simulink model "single-phase-grid-connected-inverter"  (R2020a)
settings: Solver=ode45  StartTime=0.0  StopTime=0.1  MaxStep=1e-7  MinStep=1e-8  RelTol=1e-3
libraries: powerlib x15, powerlib_meascontrol x4, simulink x1
settings Model: Creator=LENOVO PC  LastModifiedBy=User
settings SolverCC: ZeroCrossAlgorithm=Adaptive
settings DebuggingCC: IgnoredZcDiagnostic=none

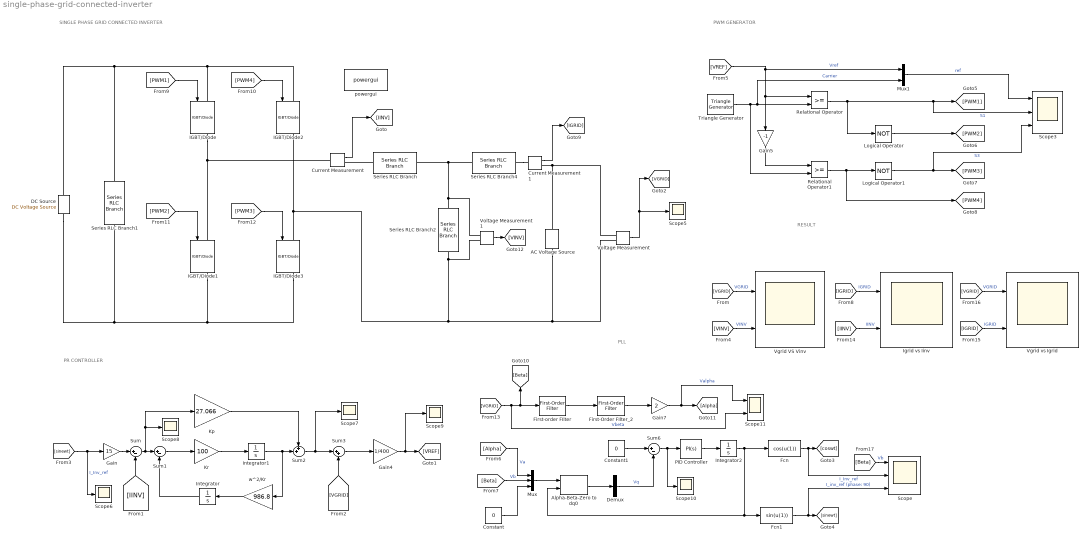
== system single-phase-grid-connected-inverter ==
  note: PR CONTROLLER
  note: SINGLE PHASE GRID CONNECTED INVERTER
  note: PWM GENERATOR
  note: PLL
  note: RESULT
  AC Voltage Source : powerlib/Electrical Sources/AC Voltage Source  Amplitude=325  Phase=0  Frequency=50  SampleTime=0  Measurements=None  BusType=swing  Pref=10e3  Qref=0  Qmin=-inf  Qmax=+inf
  Alpha-Beta-Zero to dq0 : powerlib_meascontrol/Transformations/Alpha-Beta-Zero to dq0  Alignment=90 degrees behind phase A axis
  Constant : Constant  Value=0
  Constant1 : Constant  Value=0
  Current Measurement : powerlib/Measurements/Current Measurement  PhasorSimulation=off  OutputType=Complex  PSBequivalent=0
  Current Measurement1 : powerlib/Measurements/Current Measurement  PhasorSimulation=off  OutputType=Complex  PSBequivalent=0
  DC Source : powerlib/Electrical Sources/DC Voltage Source  Amplitude=400  Measurements=None
  Demux : Demux  Outputs=3
  Fcn : Fcn  Expr=cos(u(1))
  Fcn1 : Fcn  Expr=sin(u(1))
  "First-Order FIlter_2 " : powerlib_meascontrol/Filters/First-Order Filter  FilterType=Lowpass  Tc=1/(2*pi*50)  Ts=0  Initialize=off  Vac_Init=[0, 0, 60]  Vdc_Init=0  PlotResponse=off  FreqRange="[0,  200,  1]"
  First-order FIlter : powerlib_meascontrol/Filters/First-Order Filter  FilterType=Lowpass  Tc=1/(2*pi*50)  Ts=0  Initialize=off  Vac_Init=[0, 0, 60]  Vdc_Init=0  PlotResponse=off  FreqRange="[0,  200,  1]"
  Gain : Gain  Gain=15
  Gain4 : Gain  Gain=1/400
  Gain5 : Gain  Gain=-1
  Gain7 : Gain  Gain=2
  IGBT/Diode{,1..3} (4 alike) : powerlib/Power Electronics/IGBT//Diode  Ron=1e-3  Rs=1e5  Cs=inf  Measurements=on
  Igrid vs Iinv : Scope  NumInputPorts=2
  Integrator : Integrator
  Integrator1 : Integrator
  Integrator2 : Integrator
  Kp : Gain  Gain=27.066
  Kr : Gain  Gain=100
  Logical Operator : Logic  Operator=NOT  Inputs=1  AllPortsSameDT=off  OutDataTypeStr=boolean
  Logical Operator1 : Logic  Operator=NOT  Inputs=1  AllPortsSameDT=off  OutDataTypeStr=boolean
  Mux : Mux  Inputs=3
  Mux1 : Mux  Inputs=2
  PID Controller : simulink/Continuous/PID Controller  Controller=PI  Form=Parallel  TimeDomain=Continuous-time  UseExternalTs=off  SampleTime=-1  IntegratorMethod=Forward Euler  FilterMethod=Forward Euler  ControllerParametersSource=internal  P=10  I=50000  D=0  UseFilter=on  N=100  TunerSelectOption=Transfer Function Based (PID Tuner App)  InitialConditionSource=internal  InitialConditionForIntegrator=0  InitialConditionForFilter=0  DifferentiatorICPrevScaledInput=0  ExternalReset=none  TrackingMode=off  Kt=1  LimitOutput=off  UpperSaturationLimit=inf  LowerSaturationLimit=-inf  LinearizeAsGain=on  AntiWindupMode=none  Kb=1  POutMin=[]  POutMax=[]  IOutMin=[]  IOutMax=[]  DOutMin=[]  DOutMax=[]  NOutMin=[]  NOutMax=[]  SumOutMin=[]  SumOutMax=[]  SaturationOutMin=[]  SaturationOutMax=[]  PParamMin=[]  PParamMax=[]  IParamMin=[]  IParamMax=[]  DParamMin=[]  DParamMax=[]  NParamMin=[]  NParamMax=[]  KbParamMin=[]  KbParamMax=[]  KtParamMin=[]  KtParamMax=[]  KbOutMin=[]  KbOutMax=[]  KtOutMin=[]  KtOutMax=[]  IntegratorOutMin=[]  IntegratorOutMax=[]  FilterOutMin=[]  FilterOutMax=[]  SumI1OutMin=[]  SumI1OutMax=[]  SumI2OutMin=[]  SumI2OutMax=[]  SumI3OutMin=[]  SumI3OutMax=[]  SumI4OutMin=[]  SumI4OutMax=[]  SumDOutMin=[]  SumDOutMax=[]  DifferentiatorOutMin=[]  DifferentiatorOutMax=[]  FilterDiffOutCoefMin=[]  FilterDiffOutCoefMax=[]  ReciprocalOutMin=[]  ReciprocalOutMax=[]  SumDenOutMin=[]  SumDenOutMax=[]  SumNumOutMin=[]  SumNumOutMax=[]  DivideOutMin=[]  DivideOutMax=[]  UdiffTsProdOutMin=[]  UdiffTsProdOutMax=[]  NTsProdOutMin=[]  NTsProdOutMax=[]  UintegralTsProdOutMin=[]  UintegralTsProdOutMax=[]  UngainTsProdOutMin=[]  UngainTsProdOutMax=[]  IntegratorContinuousStateAttributes=''  IntegratorStateMustResolveToSignalObject=off  IntegratorRTWStateStorageClass=Auto  FilterContinuousStateAttributes=''  FilterStateMustResolveToSignalObject=off  FilterRTWStateStorageClass=Auto  ParallelPVariant=InternalParameters  IdealPVariant=Disabled  IVariant=InternalParameters  DVariant=Disabled  IntegratorVariant=Continuous  SatVariant=Disabled  AWVariant=Passthrough  PCopyVariant=Disabled  TRVariant=Disabled  FdbkBlocksVariant=Forward  IdealPFdbkVariant=Disabled  SatFdbkVariant=Disabled  DerivativeFilterVariant=Disabled  NVariant=Disabled  NCopyVariant=Disabled_SignalSpec  FilterICVariant=Disabled  IntegratorICVariant=InternalICs  ExternalResetVariant=Disabled  TRSumVariant=Passthrough  SumFdbkVariant=Disabled  SumVariant=Sum_PI  TsampFilterVariant=InternalTs  TsampNgainVariant=Passthrough  TsampIntegralVariant=Passthrough
  Relational Operator : RelationalOperator  OutDataTypeStr=boolean  RndMeth=Simplest
  Relational Operator1 : RelationalOperator  OutDataTypeStr=boolean  RndMeth=Simplest
  Scope : Scope  NumInputPorts=3
  Scope{5..10} (6 alike) : Scope
  Scope11 : Scope  NumInputPorts=2
  Scope3 : Scope  NumInputPorts=3
  Series RLC Branch : powerlib/Elements/Series RLC Branch  LConnTagsString=__new0  RConnTagsString=__new0  BranchType=L  Resistance=0.001  Inductance=4.06e-3  SetiL0=off  InitialCurrent=0  Capacitance=1e-6  Setx0=off  InitialVoltage=0  Measurements=None
  Series RLC Branch1 : powerlib/Elements/Series RLC Branch  LConnTagsString=__new0  RConnTagsString=__new0  BranchType=RC  Resistance=0.0042  Inductance=1e-3  SetiL0=on  InitialCurrent=0  Capacitance=500e-6  Setx0=off  InitialVoltage=0  Measurements=None
  Series RLC Branch2 : powerlib/Elements/Series RLC Branch  LConnTagsString=__new0  RConnTagsString=__new0  BranchType=RC  Resistance=0.0042  Inductance=4.06e-3  SetiL0=off  InitialCurrent=0  Capacitance=6.01e-6  Setx0=off  InitialVoltage=0  Measurements=None
  Series RLC Branch4 : powerlib/Elements/Series RLC Branch  LConnTagsString=__new0  RConnTagsString=__new0  BranchType=L  Resistance=0.001  Inductance=4.35e-3  SetiL0=off  InitialCurrent=0  Capacitance=1e-6  Setx0=off  InitialVoltage=0  Measurements=None
  Sum : Sum  Inputs=|+-
  Sum1 : Sum  Inputs=|+-
  Sum2 : Sum  Inputs=++|
  Sum3 : Sum  Inputs=|++
  Sum6 : Sum  Inputs=|+-
  Triangle Generator : powerlib_meascontrol/Pulse & Signal Generators/Triangle Generator  Freq=10000  Phase=0  Ts=0
  Vgrid VS Vinv : Scope  NumInputPorts=2
  Vgrid vs Igrid : Scope  NumInputPorts=2
  Voltage Measurement : powerlib/Measurements/Voltage Measurement  PhasorSimulation=off  OutputType=Complex  PSBequivalent=0
  Voltage Measurement1 : powerlib/Measurements/Voltage Measurement  PhasorSimulation=off  OutputType=Complex  PSBequivalent=0
  powergui : powerlib/powergui  Priority=1  SimulationMode=Continuous  SampleTime=50e-6  frequency=60  Iterations=50  frequencyindice=0  Pbase=100e6  ErrMax=1e-4  UnitsV=kV  UnitsW=MW  buscounter=0  FunctionMessages=off  echomessages=off  EnableUseOfTLC=off  CurrentSourceSwitches=off  DisableSnubberDevices=off  DisableRonSwitches=off  DisableVfSwitches=off  DisplayEquations=off  AutomaticDiscreteSolvers=off  SolverType=Tustin/Backward Euler (TBE)  Interpol=off  ExternalGateDelay=off  methode=off  Ts=100  x0status=blocks  SPID=on  SwTol=0  HookPort=off  NonlinearTolerance=1e-4  nMaxIteration=100  ContinueOnMaxIteration=off  RestoreLinks=warning  ResistiveCurrentMeasurement=off  Frange=[0:2:500]  Ylog=off  Xlog=on  ShowGrid=off  save=off  variable=ZData  structure=0  ZoomFFT=off  StartTime=0.0  cycles=1  DisplayStyle=1  fundamental=60  FreqAxis=off  MaxFrequency=1000  frequencyindicesteady=1  RmsSteady=1  display=off
  w^2/Kr : Gain  Gain=986.8
  wires:
  [PWM3] -> IGBT/Diode3/1
  [PWM2] -> IGBT/Diode1/1
  [PWM1] -> IGBT/Diode/1
  [PWM4] -> IGBT/Diode2/1
  Current Measurement1/1 -> [IGRID]
  Current Measurement/1 -> [IINV]
  Voltage Measurement/1 -> Scope5/1, [VGRID]
  Sum/1 -> Scope8/1, Kp/1, Sum1/1
  Sum1/1 -> Kr/1
  Integrator1/1 -> w^2/Kr/1, Sum2/2
  Sum2/1 -> Scope7/1, Sum3/1
  [IINV] -> Sum/2
  Kr/1 -> Integrator1/1
  [VGRID] -> Sum3/2
  Gain7/1 -> Scope11/1, [Alpha]  "Valpha"
  First-order FIlter/1 -> "First-Order FIlter_2 "/1
  [VGRID] -> Scope11/2, [Beta], First-order FIlter/1  "Vbeta"
  "First-Order FIlter_2 "/1 -> Gain7/1
  Mux/1 -> Alpha-Beta-Zero to dq0/1
  Fcn/1 -> Scope/2, [coswt]  "I_Inv_ref"
  Sum6/1 -> Scope10/1, PID Controller/1
  Alpha-Beta-Zero to dq0/1 -> Demux/1
  [Beta] -> Mux/2  "Vb"
  Constant1/1 -> Sum6/1
  Integrator2/1 -> Fcn1/1, Alpha-Beta-Zero to dq0/2, Fcn/1
  PID Controller/1 -> Integrator2/1
  Constant/1 -> Mux/3
  [Alpha] -> Mux/1  "Va"
  [IGRID] -> Igrid vs Iinv/1  "IGRID"
  [sinewt] -> Scope6/1, Gain/1  "I_Inv_ref"
  Gain/1 -> Sum/1
  Sum3/1 -> Gain4/1
  Gain4/1 -> Scope9/1, [VREF]
  Demux/2 -> Sum6/2  "Vq"
  Voltage Measurement1/1 -> [VINV]
  [IINV] -> Igrid vs Iinv/2  "IINV"
  [VGRID] -> Vgrid VS Vinv/1  "VGRID"
  [VINV] -> Vgrid VS Vinv/2  "VINV"
  Kp/1 -> Sum2/1
  w^2/Kr/1 -> Integrator/1
  Integrator/1 -> Sum1/2
  Logical Operator1/1 -> Scope3/3, [PWM3]  "S3"
  Gain5/1 -> Relational Operator1/1
  Relational Operator1/1 -> Logical Operator1/1, [PWM4]
  Triangle Generator/1 -> Relational Operator1/2, Mux1/2, Relational Operator/2  "Carrier"
  [VREF] -> Mux1/1, Gain5/1, Relational Operator/1  "Vref"
  Relational Operator/1 -> Logical Operator/1, Scope3/2, [PWM1]  "S1"
  Logical Operator/1 -> [PWM2]
  Mux1/1 -> Scope3/1  "ref"
  [IGRID] -> Vgrid vs Igrid/2  "IGRID"
  [VGRID] -> Vgrid vs Igrid/1  "VGRID"
  Fcn1/1 -> Scope/3, [sinewt]  "I_inv_ref (phase: 90)"
  [Beta] -> Scope/1  "Vb"
  connections:
  Voltage Measurement/LConn1 -- AC Voltage Source/RConn1 -- Current Measurement1/RConn1
  IGBT/Diode2/LConn1 -- Series RLC Branch1/LConn1 -- DC Source/RConn1 -- IGBT/Diode/LConn1
  Series RLC Branch1/RConn1 -- DC Source/LConn1 -- IGBT/Diode3/RConn1 -- IGBT/Diode1/RConn1
  IGBT/Diode2/RConn1 -- Voltage Measurement1/LConn2 -- Series RLC Branch2/RConn1 -- Voltage Measurement/LConn2 -- AC Voltage Source/LConn1 -- IGBT/Diode3/LConn1
  Series RLC Branch2/LConn1 -- Voltage Measurement1/LConn1 -- Series RLC Branch4/LConn1 -- Series RLC Branch/RConn1
  Current Measurement/LConn1 -- IGBT/Diode/RConn1 -- IGBT/Diode1/LConn1
  Series RLC Branch/LConn1 -- Current Measurement/RConn1
  Series RLC Branch4/RConn1 -- Current Measurement1/LConn1
